simulink model "F16ASYM_Controlled_AoA"  (R2012b)
settings: Solver=ode3  SolverMode=SingleTasking  StartTime=0.0  StopTime=inf  FixedStep=T_sim  RelTol=1e-3
InitFcn:
  | load('NN_c_weights_Last_stable.mat')
values from neighbouring files (symbols this model uses):
  K_b_AoA = params(3)    [Cost_function.m]
  K_b_q = params(4)    [Cost_function.m]
  learning = 20    [Scheduling_desing.m]
  Model_used_flag = 1    [Scheduling_desing.m]
  reg_param = 0.5    [Scheduling_desing.m]
  T_sim = 0.02    [Scheduling_desing.m]
  tau_AoA = params(1)    [Cost_function.m]
  tau_q = params(2)    [Cost_function.m]
  Theta_1_roll_last = [0.00183613313267 0.00115998993235 0.0006676025148 0.00194921904952 0.00134963559861 0.00034352059664 0.000447169388141 0.00146749660935 0.00110199952389 7.77922383894e-05 0.00109492833348 0.00192687590535 ... (360 elements, 30x12)]    [NN_i_weights_LAST_STABLE.mat]
  Theta_2_roll_last = [0.000469743069697 0.000355923851088 0.00180035760697 0.00191855117771 0.00118851504447 0.0013331642065 0.0013164316578 0.000643981263341 0.00176817665434 0.000113802099363 0.000426534542462 0.00113815782354 ... (620 elements, 20x31)]    [NN_i_weights_LAST_STABLE.mat]
  Theta_3_roll_last = [9.62071520568e-05 -0.000389870886846 2.08260845013e-05 0.000140787743673 -0.000917525755397 -0.0014324207578 -0.00154701573815 -0.00131544476264 -0.00101205584381 5.06515794689e-05 -0.00111443483676 -0.00143957416141 ... (21 elements, 1x21)]    [NN_i_weights_LAST_STABLE.mat]
  V_long_lastA_w_z = [0.352826086601 -0.253633004548 -0.642535042878 0.237749930435 -0.618390629538 0.858074761295 0.268211230628 -0.448715080196 -0.0406384631192 0.401147605577 0.60598427709 0.0500551915851 ... (300 elements, 30x10)]    [NN_i_weights_LAST_STABLE.mat]
  V_long_lastAoA = [0.0774300162379 0.0911421319631 0.0352371192557 0.0542170286952 0.0651171200844 0.0177112012707 0.0982957728448 0.000259994642558 0.0194724569123 0.0466321328252 0.0556687953852 0.0252668067142 ... (300 elements, 30x10)]    [NN_i_weights_LAST_STABLE.mat]
  V_roll_last = [0.0540918675943 0.0557493347212 0.0839792276608 0.0460576391794 0.0671229058124 0.100220403067 0.0722493281881 0.0648875457457 0.00447599349201 0.0607299103823 0.0488037966361 0.0176785979393 ... (360 elements, 30x12)]    [NN_i_weights_LAST_STABLE.mat]
  V_yaw_last = [0.0965149149679 0.00833616709545 0.0365734360076 0.0523944217566 0.00790252078455 0.0700053845887 0.0345164868709 0.0111568465295 0.094060639546 0.0205483560006 0.000798047494256 0.0862769385758 ... (360 elements, 30x12)]    [NN_i_weights_LAST_STABLE.mat]
  velocity = M_eval_sche(I,J)*a    [Scheduling_desing.m]
  W_long_lastA_w_z = [-0.0522913429974 0.00385484301394 -0.00465489482472 -0.0139416219936 0.00295196421483 -0.013027768541 0.00585545058915 0.00278802233571 -0.00906272782329 -0.000396112031465 0.00405849743321 0.00509668457818 ... (31 elements, 1x31)]    [NN_i_weights_LAST_STABLE.mat]
  W_long_lastAoA = [-0.0192589013922 0.00873109909713 0.00432649597332 0.0420946902441 0.0293366820194 0.0351497798191 0.0234952374236 0.0360841187718 0.0112233388211 0.030147202199 0.0369533138617 0.00218839076415 ... (31 elements, 1x31)]    [NN_i_weights_LAST_STABLE.mat]
  W_roll_last = [-0.0006515532842 0.000535485585715 0.000550946920743 0.000806030945453 0.00045976209382 0.00065557954304 0.000945902185602 0.00070191398535 0.000635215543728 4.66501377412e-05 0.000597079583757 0.000485790566765 ... (31 elements, 1x31)]    [NN_i_weights_LAST_STABLE.mat]
  W_yaw_last = [-4.34263633305e-05 8.83823048922e-05 1.65575463724e-05 3.60293102233e-05 5.19752447623e-05 7.06399280852e-06 7.02425975821e-05 3.62680255076e-05 1.29996379937e-05 8.05072914397e-05 2.39941870661e-05 2.52427840574e-06 ... (31 elements, 1x31)]    [NN_i_weights_LAST_STABLE.mat]
undefined symbols (not defined in the file or in its folder): a1, alpha_map_eval, B, beta_map_eval, C_L_0, DiscIntNeverNeededParam, fi_flag_Simulink, G_eval, H_sq, H_sq_autotrim, k_B, m_B, M_sq, M_sq_autotrim, sigbuilder_block, Stall_curve, trim_control, trim_state, trim_throttle, V_Comp_A_w_z_last, V_Comp_last, V_roll_lastMOD, W_Comp_A_w_z_last, W_Comp_last, W_roll_lastMOD
libraries: Adaptive_FaultTolerantControl x43, dspsigops x29, F16_Actuator_Library x14, simulink x8, aerolibatmos2 x7, dsparch4 x6, simulink_extras x5, aerolibtransform2 x5, qcatlib x4, dspmtrx3 x3, dspvision x2, dspsnks4 x2
(part 2 of 11)

== system F16ASYM_Controlled_AoA/Anti-windup Calculation/Anti-windup: Reconfigurable ==
  note: INPUTS
      | States:
      |
      | 1. Altitude
      | 2. TAS velocity
      | 3. alpha in rad
      | 4. beta in rads
      | 5. P
      | 6. Q
      | 7. R
      | 8. Throttle
      | 9. Elevator_L in deg
      | 10. Elevator_R in deg
      | 11. Aileron_L
      | 12. Aileron_R
      | 13. Rudder
      | 14. LEF_L
      | 15. LEF_R
      |
      | RECONFIGURATION PARAMETERS
      |
      | 16. mass  Estimated mass
      | 17. S_current_L
      | 18. S_current_R
      | 19. S_fin_current
      | 20. x_cg
      | 21. Jy
      | 22. Jxz
      | 23. Jz
      | 24. Jx
      | 25. EFF_el_L
      | 26. EFF_el_R
      | 27. EFF_ail_L
      | 28 EFF_ail_R
      | 29. EFF_rud
      | 30. EFF_lef_L
      | 31. EFF_lef_R
      | 32. Delta_C_Lift_X
      | 33. Delta_C_Drag_X
      | 34. Delta_C_m_X
  note: Reached Angular accel
  note: Converto to Angular accelerations
  Ang accel comm : Inport
  Est reconf : Inport  Port=2
  All_meas : Inport  Port=3
  Surf saturated : Inport  Port=4
  Control_defl : Inport  Port=5
  AWU signals : Scope
      settings: YMin=-2.5  YMax=4.5  SaveName=ScopeData7
  AWU signals1 : Scope
      settings: YMin=-3.5  YMax=1.5  SaveName=ScopeData12
  Analog Filter Design1 : dsparch4/Analog Filter Design  method=Butterworth  filttype=Lowpass  N=8  Wlo=2*pi/T_sim/5  Whi=80  Rp=2  Rs=40
  Analog Filter Design2 : dsparch4/Analog Filter Design  method=Butterworth  filttype=Lowpass  N=8  Wlo=2*pi/T_sim/5  Whi=80  Rp=2  Rs=40
  Analog Filter Design3 : dsparch4/Analog Filter Design  method=Butterworth  filttype=Lowpass  N=8  Wlo=2*pi/T_sim/5  Whi=80  Rp=2  Rs=40
  Ang Accel : MATLAB Function
  Antiwindup calculation : MATLAB Function  TreatAsAtomicUnit=on
  Bus Selector : BusSelector  OutputSignals=signal1.Alt meas (m),signal1.V_TAS (m/s),signal1.AoA meas (rad),signal1.SS meas (rad),signal1.omega_b meas (rad/s),signal1.Throttle_meas
  Bus Selector1 : BusSelector  OutputSignals=signal2.q (Pa),signal1.omega_b meas (rad/s)
  Bus Selector2 : BusSelector  OutputSignals=Reconfig signal
  Demux : Demux  Outputs=3
  Demux1 : Demux  Outputs=3
  Effectiveness Matrix B : Constant  Value=B
  Memory1 : Memory  X0=[0,0,0]
  "Mom coefficients that can was reached " : MATLABFcn  MATLABFcn=Moms_Coeff_Reconf_estimator  OutputDimensions=3  OutputSignalType=real
  Moments : Subsystem
  Mux : Mux  Inputs=3
  Mux1 : Mux  Inputs=7
  Mux2 : Mux  Inputs=3
  Mux3 : Mux  Inputs=[15 19]
  Selector : Selector  InputPortWidth=8  IndexOptions=Index vector (dialog)  Indices=1:7  OutputSizes=1
  Signal Specification : SignalSpecification  Dimensions=19
  Transfer Fcn1 : TransferFcn  Commented=on  Numerator=10  Denominator=[1 10]
  Anti-windup signals : Outport
  wires:
  Bus Selector/6 -> Mux1/6  "<Throttle_meas>"
  Control_defl/1 -> Selector/1
  Bus Selector/4 -> Mux1/4  "<SS meas (rad)>"
  Bus Selector/3 -> Mux1/3  "<AoA meas (rad)>"
  Bus Selector/2 -> Mux1/2  "<V_TAS (m/s)>"
  Bus Selector/1 -> Mux1/1  "<Alt meas (m)>"
  Bus Selector/5 -> Mux1/5  "<omega_b meas (rad/s)>"
  Selector/1 -> Antiwindup calculation/5(deflections), Mux1/7
  Est reconf/1 -> Bus Selector2/1
  Bus Selector2/1 -> Signal Specification/1  "<Reconfig signal>"
  Mux1/1 -> Mux3/1
  Mux3/1 -> "Mom coefficients that can was reached "/1
  Signal Specification/1 -> Mux3/2
  All_meas/1 -> Bus Selector1/1, Bus Selector/1
  Ang Accel/2(q_dot) -> Mux/2
  Ang Accel/3(r_dot) -> Mux/3
  Ang Accel/1(p_dot) -> Mux/1
  Bus Selector1/2 -> Ang Accel/4(omega_b)  "<omega_b meas (rad/s)>"
  Moments/3(N) -> Ang Accel/3(N)
  Moments/2(M) -> Ang Accel/2(M)
  Moments/1(L) -> Ang Accel/1(L)
  Bus Selector1/1 -> Moments/4(q)  "<q (Pa)>"
  Demux/3 -> Moments/3(C_N)
  Demux/2 -> Moments/2(C_M)
  Demux/1 -> Moments/1(C_L)
  "Mom coefficients that can was reached "/1 -> Demux/1
  Mux/1 -> Antiwindup calculation/2(Ang_acell_achieved)
  Effectiveness Matrix B/1 -> Antiwindup calculation/4(B)
  Surf saturated/1 -> Antiwindup calculation/3(Saturations)
  Ang accel comm/1 -> Memory1/1
  Memory1/1 -> Antiwindup calculation/1(Ang_acell_comm)
  Antiwindup calculation/1(AWU) -> Demux1/1, AWU signals/1
  Demux1/1 -> Analog Filter Design3/1
  Demux1/2 -> Analog Filter Design1/1
  Analog Filter Design3/1 -> Mux2/1
  Analog Filter Design1/1 -> Mux2/2
  Analog Filter Design2/1 -> Mux2/3
  Demux1/3 -> Analog Filter Design2/1
  Mux2/1 -> AWU signals1/1, Anti-windup signals/1

== system F16ASYM_Controlled_AoA/Auto-trim, saturations sensibility and pilot help/Command A_w_z  or  A_gamma_z ==
  note: Pass this one if >0.5
  All meas : Inport
  Acc command : Inport  Port=2
  A_b : Product  Multiplication=Matrix(*)
  A_w : Product  Multiplication=Matrix(*)
  Bus Selector3 : BusSelector  OutputSignals=signal2.T_F_b->F_T,signal2.T_F_b->F_w
  Criteria : Constant  Value=Criteria
  Gain : Gain  Gain=[0;0;-1]
  Gain1 : Gain  Gain=-1
  Selector : Selector  InputPortWidth=3  IndexOptions=Index vector (dialog)  Indices=3  OutputSizes=1
  Switch : Switch  Threshold=0.5
  Transpose : dspmtrx3/Transpose  Hermitian=off  overflowFlag=off
  A_w_z : Outport
  wires:
  All meas/1 -> Bus Selector3/1
  Criteria/1 -> Switch/2
  Acc command/1 -> Switch/3, Gain/1
  Switch/1 -> A_w_z/1
  Bus Selector3/1 -> Transpose/1  "<T_F_b->F_T>"
  Transpose/1 -> A_b/1
  Gain/1 -> A_b/2
  Bus Selector3/2 -> A_w/1  "<T_F_b->F_w>"
  A_b/1 -> A_w/2
  A_w/1 -> Selector/1
  Selector/1 -> Gain1/1
  Gain1/1 -> Switch/1

== system F16ASYM_Controlled_AoA/Cockpit/Joystick ==
  Add1 : Sum
  Add2 : Sum
  Aileron : Selector  InputPortWidth=2  IndexOptions=Index vector (dialog)  Indices=1  OutputSizes=1
  Gain : Gain  Gain=0.01  OutDataTypeStr=double
  Gain{1..2,4,8} (4 alike) : Gain
  Gain3 : Gain  Gain=-1
  Gain5 : Gain  Gain=-10
  Gain6 : Gain  Gain=10  OutDataTypeStr=double
  Gain7 : Gain  Gain=-1
  Integrator Limited2 : Integrator  LimitOutput=on  UpperSaturationLimit=400  LowerSaturationLimit=-400
  Integrator Limited3 : Integrator  LimitOutput=on  UpperSaturationLimit=1  LowerSaturationLimit=-1
  Joystick Input : vrlib/Joystick Input  joyid=1  adjustports=on  forcefeed=off
  Manual Switch : ManualSwitch
  Selector1 : Selector  InputPortWidth=5  IndexOptions=Index vector (dialog)  Indices=1:2  OutputSizes=1
  Selector2 : Selector  InputPortWidth=5  IndexOptions=Index vector (dialog)  Indices=3  OutputSizes=1
  Selector3 : Selector  InputPortWidth=5  IndexOptions=Index vector (dialog)  Indices=4:5  OutputSizes=1
  Selector4 : Selector  InputPortWidth=10  IndexOptions=Index vector (dialog)  Indices=1  OutputSizes=1
  Selector5 : Selector  InputPortWidth=10  IndexOptions=Index vector (dialog)  Indices=4  OutputSizes=1
  Selector6 : Selector  InputPortWidth=10  IndexOptions=Index vector (dialog)  Indices=1  OutputSizes=1
  Selector7 : Selector  InputPortWidth=10  IndexOptions=Index vector (dialog)  Indices=4  OutputSizes=1
  elev : Selector  InputPortWidth=2  IndexOptions=Index vector (dialog)  Indices=2  OutputSizes=1
  speed des : Outport
  Throttle : Outport  Port=2
  Long: Acc : Outport  Port=3
  Roll : Outport  Port=4
  sideslip : Outport  Port=5
  wires:
  Integrator Limited3/1 -> Throttle/1  "Throttle"
  Aileron/1 -> Gain1/1
  Manual Switch/1 -> Aileron/1, elev/1
  Joystick Input/1 -> Selector2/1, Selector3/1, Selector1/1
  Selector1/1 -> Manual Switch/1
  Selector3/1 -> Manual Switch/2
  Selector4/1 -> Gain3/1
  Selector5/1 -> Gain4/1
  Gain3/1 -> Add1/1
  Gain4/1 -> Add1/2
  Add1/1 -> Gain/1
  Gain/1 -> Integrator Limited3/1
  elev/1 -> Gain2/1
  Gain1/1 -> Roll/1
  Selector2/1 -> Gain5/1
  Gain2/1 -> Long: Acc/1
  Gain5/1 -> sideslip/1
  Integrator Limited2/1 -> speed des/1  "Throttle"
  Joystick Input/2 -> Selector5/1, Selector7/1, Selector6/1, Selector4/1
  Selector6/1 -> Gain7/1
  Selector7/1 -> Gain8/1
  Gain7/1 -> Add2/1
  Gain8/1 -> Add2/2
  Add2/1 -> Gain6/1
  Gain6/1 -> Integrator Limited2/1

== system F16ASYM_Controlled_AoA/Cockpit/Signal Builder1 ==
  Demux : Demux  Tag=STV Demux
  FromWs : FromWorkspace  Tag=STV FromWs  VariableName=tuvar  SampleTime=0
      SigBuilderData=|
      | common.afterFinalStr = 'Extrapolate'
      | common.sampleTime = 0
      | dataSet.timeRange = [0 30]
      | dataSet.name = 'Group 1'
      | sbobj.Groups.Name = 'Group 1'
      | sbobj.Groups.Signals(1).Name = 'Signal 1'
      | sbobj.Groups.Signals(1).XData = [0 0.5 0.5 2.5 2.5 30]
      | sbobj.Groups.Signals(1).YData = [0 0 -1 -1 0 0]
      | sbobj.Groups.Signals(2).Name = 'Signal 5'
      | sbobj.Groups.Signals(2).XData = [0 4 4 6 6 30]
      | sbobj.Groups.Signals(2).YData = [0 0 1 1 0 0]
      | sbobj.Groups.Signals(3).Name = 'Signal 6'
      | sbobj.Groups.Signals(3).XData = [0 8 8 10 10 30]
      | sbobj.Groups.Signals(3).YData = [0 0 -0.5 -0.5 0 0]
      | sbobj.Groups.Signals(4).Name = 'Signal 7'
      | sbobj.Groups.Signals(4).XData = [0 12 12 14 14 30]
      | sbobj.Groups.Signals(4).YData = [0 0 0.5 0.5 0 0]
      | sbobj.Groups.TimeRange = [0 30]
  Signal 1 : Outport  Tag=STV Outport
  Signal 5 : Outport  Tag=STV Outport  Port=2
  Signal 6 : Outport  Tag=STV Outport  Port=3
  Signal 7 : Outport  Tag=STV Outport  Port=4
  wires:
  FromWs/1 -> Demux/1
  Demux/1 -> Signal 1/1
  Demux/2 -> Signal 5/1
  Demux/3 -> Signal 6/1
  Demux/4 -> Signal 7/1

== system F16ASYM_Controlled_AoA/Cockpit/Signal Builder2 ==
  Demux : Demux  Tag=STV Demux
  FromWs : FromWorkspace  Tag=STV FromWs  VariableName=tuvar  SampleTime=0
      SigBuilderData=|
      | common.afterFinalStr = 'Extrapolate'
      | common.sampleTime = 0
      | dataSet.timeRange = [0 10]
      | dataSet.name = 'Group 1'
      | sbobj.Groups.Name = 'Group 1'
      | sbobj.Groups.Signals(1).Name = 'Signal 1'
      | sbobj.Groups.Signals(1).XData = [0 5 5 8.02 8.02 10]
      | sbobj.Groups.Signals(1).YData = [0 0 -8.15 -8.15 0.64 0.7]
      | sbobj.Groups.Signals(2).Name = 'Signal 2'
      | sbobj.Groups.Signals(2).XData = [0 10]
      | sbobj.Groups.Signals(2).YData = [0 0]
      | sbobj.Groups.Signals(3).Name = 'Signal 3'
      | sbobj.Groups.Signals(3).XData = [0 10]
      | sbobj.Groups.Signals(3).YData = [0 0]
      | sbobj.Groups.Signals(4).Name = 'Signal 4'
      | sbobj.Groups.Signals(4).XData = [0 10]
      | sbobj.Groups.Signals(4).YData = [0 0]
  Signal 1 : Outport  Tag=STV Outport
  Signal 2 : Outport  Tag=STV Outport  Port=2
  Signal 3 : Outport  Tag=STV Outport  Port=3
  Signal 4 : Outport  Tag=STV Outport  Port=4
  wires:
  FromWs/1 -> Demux/1
  Demux/1 -> Signal 1/1
  Demux/2 -> Signal 2/1
  Demux/3 -> Signal 3/1
  Demux/4 -> Signal 4/1

== matlab function F16ASYM_Controlled_AoA/Anti-windup Calculation/Anti-windup: NO reconfigurable/Antiwindup calculation ==
  data: Ang_acell_comm input; AWU output; Ang_acell_achieved input; Saturations input; B input; deflections input
function AWU = AWU_calculation(Ang_acell_comm,Ang_acell_achieved,Saturations,B,deflections)
% Computing Saturation limits
sup_limit = [24,24,21,21,29,25,25]-1;
inf_limit = [-24,-24,-21,-21,-29,0,0]+1;

for i=1:7
    Saturations(i) = Saturation_smooth(abs(Saturations(i)),deflections(i),sup_limit(i),inf_limit(i));
end
Sat_B = B*Saturations;
B_max = B*ones(7,1);

AWU=zeros(3,1);

%% Method A
% % psi = 0.01; % % of the effort above the one we consider manouvreability is reduced
% % for i=1:3
% %     if i==1 && sign(deflections(3))== sign(deflections(4)) && abs(Sat_B(i))>psi*abs(B_max(i))
% %         AWU(2) = Ang_acell_comm(2) - Ang_acell_achieved(2); % we have to desaturate longitudinally not laterally
% %     elseif  i==1 && sign(deflections(3))~= sign(deflections(4)) && abs(Sat_B(i))>psi*abs(B_max(i))
% %         AWU(i) = Ang_acell_comm(i) - Ang_acell_achieved(i);
% %     elseif i~=1 && abs(Sat_B(i))>psi*abs(B_max(i))
% %         AWU(i) = Ang_acell_comm(i) - Ang_acell_achieved(i);
% %     end 
% % end

%% Method B
% % % % Long
% % % if Saturations(1)~=0 || Saturations(2)~=0 ||  Saturations(6)~=0 || Saturations(7)~=0 || ((Saturations(3)~=0 || Saturations(4)~=0) && sign(deflections(3))== sign(deflections(4)) ) 
% % %     AWU(2) = Ang_acell_comm(2) - Ang_acell_achieved(2);
% % % end
% % % % Lat-dir
% % % if ((Saturations(3)~=0 || Saturations(4)~=0) && sign(deflections(3)) ~= sign(deflections(4)) )  || Saturations(5)~=0 || Saturations(6)~=0 || Saturations(7)~=0
% % %     AWU(1) = Ang_acell_comm(1) - Ang_acell_achieved(1);
% % %     AWU(3) = Ang_acell_comm(3) - Ang_acell_achieved(3);
% % % 
% % % end



%% Method C
for i=1:3
        AWU(i) = (Ang_acell_comm(i) - Ang_acell_achieved(i))*Sat_B(i)/norm(B(i,:));
end

end

function Saturation_out = Saturation_smooth(Saturation,angle,sup_limit,inf_limit)

a=5;
Saturation_out  = ( 1 - 1./(1+exp(-a*(angle-inf_limit ))) + 1./(1+exp(-a*(angle-sup_limit ))) )*Saturation;


end

== matlab function F16ASYM_Controlled_AoA/Primary Controller/P  + Crossed NN + AWU+Lim + hand-over/P controller + adaptive Crossed NN + AWU+Lim   in AoA/Physical limitation/Ang Accel ==
  data: L input; p_dot output; q_dot output; r_dot output; M input; N input; omega_b input
function [p_dot,q_dot,r_dot] = Ang_accel(L,M,N,omega_b)
Jy  = 75673.6;
Jxz = 1331.4; 
Jz  = 85552.1;  
Jx  = 12874.8;
h_E = 216.9;

denom = Jx*Jz - Jxz*Jxz;

% % C1 = ((Jy - Jz)  * Jz  - (Jxz * Jxz))/ Gamma;
% % C2 = ((Jx - Jy + Jz ) * Jxz ) / Gamma;
% % C3 = Jz / Gamma;
% % C4 = Jxz / Gamma;
% % C5 = (Jz - Jx) / Jy;
% % C6 = Jxz / Jy ;
% % C7 = 1 / Jy;
% % C8 = (Jx * (Jx - Jy ) + Jxz * Jxz) / Gamma;
% % C9 = Jx / Gamma;


p_dot =  (Jz*L + Jxz*N - (Jz*(Jz-Jy)+Jxz*Jxz)*omega_b(2)*omega_b(3) + Jxz*(Jx-Jy+Jz)*omega_b(1)*omega_b(2) + Jxz*omega_b(2)*h_E)/denom;

q_dot = (M + (Jz-Jx)*omega_b(1)*omega_b(3) - Jxz*(omega_b(1)*omega_b(1)-omega_b(3)*omega_b(3)) - omega_b(3)*h_E)/Jy;


r_dot = (Jx*N + Jxz*L + (Jx*(Jx-Jy)+Jxz*Jxz)*omega_b(1)*omega_b(2) - Jxz*(Jx-Jy+Jz)*omega_b(2)*omega_b(3) +  Jx*omega_b(2)*h_E)/denom;

== matlab function F16ASYM_Controlled_AoA/Primary Controller/P  + Crossed NN + AWU+Lim + hand-over/P controller + adaptive Crossed NN + AWU+Lim    in ACC /Physical limitation/max deflections estimator ==
  data: v_comm input; max_defl output; B parameter
function max_defl = Max_defl(v_comm,B)
sup_limit = [24,24,21,21,29,25,25];
inf_limit = [-24,-24,-21,-21,-29,0,0];

def=B;
for i=1:3
    def(i,:) = B(i,:).*sign(v_comm(i));
end
def_avg = mean(def,1);

max_defl = zeros(7,1);
for i=1:7
    if def_avg(1,i)>0
        max_defl(i) = sup_limit(i);
    else
        max_defl(i) = inf_limit(i);
    end
end

== matlab function F16ASYM_Controlled_AoA/P controller + adaptive Crossed NN + AWU+Lim+scheduling   in AoA/Physical limitation/max deflections estimator ==
  data: v_comm input; max_defl output; B parameter
function max_defl = Max_defl(v_comm,B)
sup_limit = [24,24,21,21,29,25,25];
inf_limit = [-24,-24,-21,-21,-29,0,0];

def=B;
for i=1:3
    def(i,:) = B(i,:).*sign(v_comm(i));
end
def_avg = mean(def,1);

max_defl = zeros(7,1);
for i=1:7
    if def_avg(1,i)>0
        max_defl(i) = sup_limit(i);
    else
        max_defl(i) = inf_limit(i);
    end
end

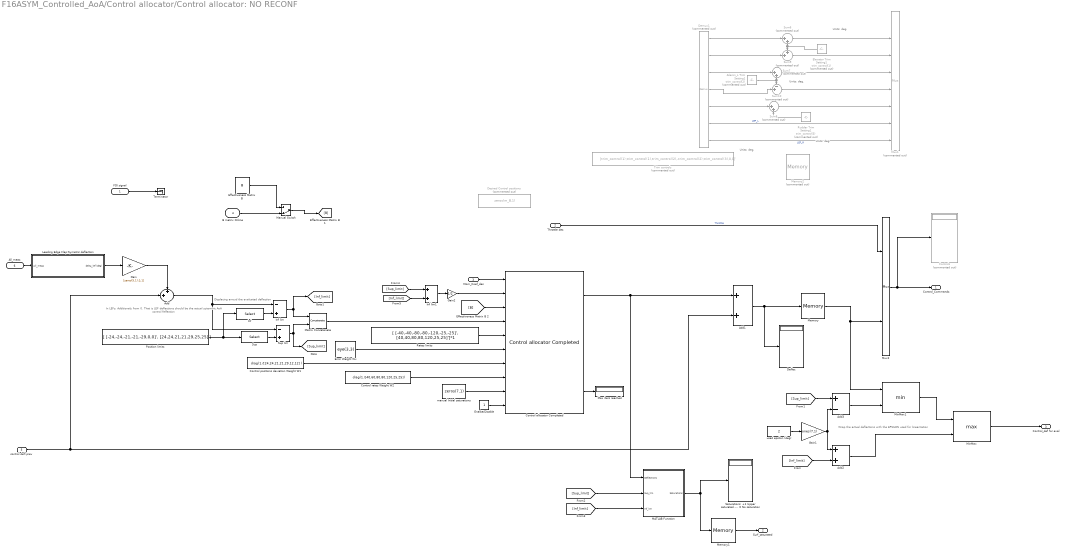
== system F16ASYM_Controlled_AoA/Control allocator/Control allocator: NO RECONF ==
  note: Wrap the actual deflections with the EPSILON
      |  used for linearization
  note: Units: deg.
  note: Units: deg.
  note: Units: deg.
  note: Units: deg.
  note: In LEFs: Additionaly from 0.  That is LEF deflections should be
      | the actual sytemtric AoA control felfection
  note: Displacing arroud the evaluated deflection
  FDI signal : Inport
  Throttle des : Inport  Port=2
  Mom_Coef_des : Inport  Port=3
  B matrix Online : Inport  Port=4
  control defl prev : Inport  Port=5
  All_meas : Inport  Port=6
  Add : Sum  Inputs=++|
  Add1 : Sum
  Add2 : Sum
  Add3 : Sum  Inputs=+-
  Aileron_L Trim Setting1 : Constant  Commented=on  Value=trim_control(2)
  "Control allocator Completed " : qcatlib/Control allocator Completed   alg=SLS  CA_type=QP  iter_max=100  gamma=1e6  k_B=3  m_B=7  T=T_sim  tol=1e-5
  Control positions deviation Weight W1 : Constant  Value=diag(1./[24,24,21,21,29,12,12] )
  Control rates Weight W2 : Constant  Value=diag(1./[40,60,80,80,120,25,25])
  Controls : Display  Commented=on
  Deflec : Display
  Demux1 : Demux  Commented=on  Outputs=[1,1,1,1,1,1,1]
  Desired Control positions : Constant  Commented=on  Value=zeros(m_B,1)
  Effectiveness Matrix B : Constant  Value=B
  Elevator Trim Setting1 : Constant  Commented=on  Value=trim_control(1)  VectorParams1D=off
  Enalbe/Disable : Constant
  Error Weight Wv : Constant  Value=eye(3,3)
  Gain : Gain  Gain=[zeros(5,1);1;1]
  Gain1 : Gain  Gain=ones(7,1)
  Gain2 : Gain  Gain=1/2
  Inf : Selector  NumberOfDimensions=2  InputPortWidth=3  IndexOptions=Index vector (dialog),Index vector (dialog)  Indices=[1:7],1  OutputSizes=1,1
  Inf lim : Sum  Inputs=-+
  Inf lim1 : Sum
  Leading Edge Flap:Symetric deflection : Subsystem
  MATLAB Function : MATLAB Function  TreatAsAtomicUnit=on
  Manual Switch : ManualSwitch  CurrentSetting=0
  Matrix Concatenate : Concatenate  Mode=Multidimensional array  ConcatenateDimension=2
  Max iters reached : Display
  Memory : Memory  X0=[trim_control(1),trim_control(1),trim_control(2),-trim_control(2),trim_control(3),0,0]'
  Memory1 : Memory  X0=zeros(7,1)
  Memory2 : Memory  Commented=on  X0=zeros(7,1)
  MinMax : MinMax  Function=max  Inputs=2
  MinMax1 : MinMax  Inputs=2
  Mux1 : Mux  Commented=on  Inputs=8
  Mux2 : Mux  Inputs=[1 7]
  Position limits : Constant  Value=[ [-24,-24,-21,-21,-29,0,0]', [24,24,21,21,29,25,25]']
  Rates limits : Constant  Value=[ [-40,-40,-80,-80,-120,-25,-25]', [40,40,80,80,120,25,25]']*1
  Rudder Trim Setting1 : Constant  Commented=on  Value=trim_control(3)
  Saturations: +1 Upper saturated -1 Lower saturated 0 No saturation : Display
  Sum10 : Sum  Commented=on  Inputs=-+|  SaturateOnIntegerOverflow=on  InputSameDT=on  OutDataTypeStr=Inherit: Same as first input
  Sum6 : Sum  Commented=on  Inputs=|++  SaturateOnIntegerOverflow=on  InputSameDT=on  OutDataTypeStr=Inherit: Same as first input
  Sum7 : Sum  Commented=on  Inputs=|++  SaturateOnIntegerOverflow=on  InputSameDT=on  OutDataTypeStr=Inherit: Same as first input
  Sum8 : Sum  Commented=on  Inputs=|++  SaturateOnIntegerOverflow=on  InputSameDT=on  OutDataTypeStr=Inherit: Same as first input
  Sum9 : Sum  Commented=on  Inputs=++|  SaturateOnIntegerOverflow=on  InputSameDT=on  OutDataTypeStr=Inherit: Same as first input
  Sup : Selector  NumberOfDimensions=2  InputPortWidth=3  IndexOptions=Index vector (dialog),Index vector (dialog)  Indices=[1:7],2  OutputSizes=1,1
  Sup lim : Sum  Inputs=-+
  Terminator : Terminator
  "Trim controls " : Constant  Commented=on  Value=[trim_control(1),trim_control(1),trim_control(2),-trim_control(2),trim_control(3),0,0]'
  manual Initial saturations : Constant  Value=zeros(7,1)
  used epsilon (deg) : Constant  Value=2
  Control_Commands : Outport
  Surf_saturated : Outport  Port=2
  Control_def for eval : Outport  Port=3
  wires:
  MinMax/1 -> Control_def for eval/1
  MinMax1/1 -> MinMax/1
  Add3/1 -> MinMax1/2
  used epsilon (deg)/1 -> Gain1/1
  [Inf_limit] -> Add2/2
  Gain1/1 -> Add3/2, Add2/1
  [Sup_limit] -> Add3/1
  Add2/1 -> MinMax/2
  Memory/1 -> Mux2/2, MinMax1/1
  Add1/1 -> Memory/1, Deflec/1
  Demux1/5 -> Sum8/1
  Rudder Trim Setting1/1 -> Sum8/2
  Elevator Trim Setting1/1 -> Sum9/1, Sum6/2
  Demux1/4 -> Sum10/2
  Demux1/3 -> Sum7/1
  Demux1/2 -> Sum9/2
  Demux1/1 -> Sum6/1
  Demux1/7 -> Mux1/8  "LEF_R"
  Demux1/6 -> Mux1/7  "LEF_L"
  Sum9/1 -> Mux1/3
  Sum6/1 -> Mux1/2
  Aileron_L Trim Setting1/1 -> Sum10/1, Sum7/2
  Sum10/1 -> Mux1/5
  Sum8/1 -> Mux1/6
  Sum7/1 -> Mux1/4
  ? -> Mux1/1  "Throttle"
  Control positions deviation Weight W1/1 -> "Control allocator Completed "/7
  FDI signal/1 -> Terminator/1
  Leading Edge Flap:Symetric deflection/1(delta_lef (deg)) -> Gain/1
  All_meas/1 -> Leading Edge Flap:Symetric deflection/1(All_meas)
  Gain/1 -> Add/1
  control defl prev/1 -> Add1/2, Add/2
  Manual Switch/1 -> [B]
  Effectiveness Matrix B/1 -> Manual Switch/1
  B matrix Online/1 -> Manual Switch/2
  "Control allocator Completed "/1 -> MATLAB Function/1(Deflections), Add1/1
  Enalbe/Disable/1 -> "Control allocator Completed "/10
  manual Initial saturations/1 -> "Control allocator Completed "/9
  "Control allocator Completed "/3 -> Max iters reached/1
  [B] -> "Control allocator Completed "/3
  Sup lim/1 -> [Sup_limit], Matrix Concatenate/2
  Inf lim/1 -> [Inf_limit], Matrix Concatenate/1
  Matrix Concatenate/1 -> "Control allocator Completed "/4
  Inf/1 -> Inf lim/2
  Add/1 -> Inf lim/1, Sup lim/1
  Sup/1 -> Sup lim/2
  Control rates Weight W2/1 -> "Control allocator Completed "/8
  Error Weight Wv/1 -> "Control allocator Completed "/6
  Rates limits/1 -> "Control allocator Completed "/5
  Position limits/1 -> Sup/1, Inf/1
  Gain2/1 -> "Control allocator Completed "/2
  Mux2/1 -> Control_Commands/1, Controls/1
  Throttle des/1 -> Mux2/1  "Throttle"
  Mom_Coef_des/1 -> "Control allocator Completed "/1
  [Sup_limit] -> MATLAB Function/2(Sup_lim)
  [Inf_limit] -> MATLAB Function/3(Inf_lim)
  MATLAB Function/1(Saturations) -> Memory1/1, Saturations: +1 Upper saturated -1 Lower saturated 0 No saturation/1
  [Sup_limit] -> Inf lim1/1
  [Inf_limit] -> Inf lim1/2
  Inf lim1/1 -> Gain2/1
  Memory1/1 -> Surf_saturated/1

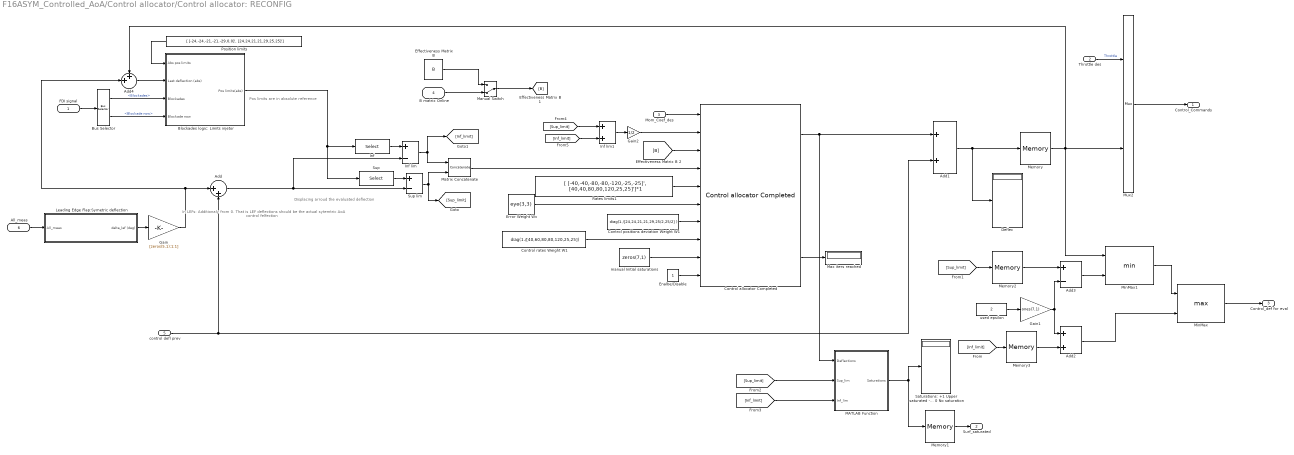
== system F16ASYM_Controlled_AoA/Control allocator/Control allocator: RECONFIG ==
  note: Pos limits are in absolute reference
  note: In LEFs: Additionaly from 0.  That is LEF deflections should be
      | the actual sytemtric AoA control felfection
  note: Displacing arroud the evaluated deflection
  FDI signal : Inport
  Throttle des : Inport  Port=2
  Mom_Coef_des : Inport  Port=3
  B matrix Online : Inport  Port=4
  control defl prev : Inport  Port=5
  All_meas : Inport  Port=6
  Add : Sum  Inputs=|++
  Add1 : Sum
  Add2 : Sum
  Add3 : Sum  Inputs=+-
  Add4 : Sum  Inputs=++|
  Blockades logic: Limits injetor : Subsystem
  Bus Selector : BusSelector  OutputSignals=Blockades,Blockade now
  "Control allocator Completed " : qcatlib/Control allocator Completed   alg=WLS  CA_type=QP  iter_max=100  gamma=1e8  k_B=3  m_B=7  T=T_sim  tol=1e-5
  Control positions deviation Weight W1 : Constant  Value=diag(1./[24,24,21,21,29,25/2,25/2] )
  Control rates Weight W1 : Constant  Value=diag(1./[40,60,80,80,120,25,25])
  Deflec : Display
  Effectiveness Matrix B : Constant  Value=B
  Enalbe/Disable : Constant
  Error Weight Wv : Constant  Value=eye(3,3)
  Gain : Gain  Gain=[zeros(5,1);1;1]
  Gain1 : Gain  Gain=ones(7,1)
  Gain2 : Gain  Gain=1/2
  Inf : Selector  NumberOfDimensions=2  InputPortWidth=3  IndexOptions=Index vector (dialog),Index vector (dialog)  Indices=[1:7],1  OutputSizes=1,1
  Inf lim : Sum  Inputs=+-
  Inf lim1 : Sum
  Leading Edge Flap:Symetric deflection : Subsystem
  MATLAB Function : MATLAB Function  TreatAsAtomicUnit=on
  Manual Switch : ManualSwitch  CurrentSetting=0
  Matrix Concatenate : Concatenate  Mode=Multidimensional array  ConcatenateDimension=2
  Max iters reached : Display
  Memory : Memory  X0=[trim_control(1),trim_control(1),trim_control(2),-trim_control(2),trim_control(3),0,0]'
  Memory1 : Memory  X0=zeros(7,1)
  Memory2 : Memory  X0=[24,24,21,21,29,25,25]'
  Memory3 : Memory  X0=[-24,-24,-21,-21,-29,0,0]'
  MinMax : MinMax  Function=max  Inputs=2
  MinMax1 : MinMax  Inputs=2
  Mux2 : Mux  Inputs=[1 7]
  Position limits : Constant  Value=[ [-24,-24,-21,-21,-29,0,0]', [24,24,21,21,29,25,25]']
  Rates limits1 : Constant  Value=[ [-40,-40,-80,-80,-120,-25,-25]', [40,40,80,80,120,25,25]']*1
  Saturations: +1 Upper saturated -1 Lower saturated 0 No saturation : Display
  Sup : Selector  NumberOfDimensions=2  InputPortWidth=3  IndexOptions=Index vector (dialog),Index vector (dialog)  Indices=[1:7],2  OutputSizes=1,1
  Sup lim : Sum  Inputs=+-
  manual Initial saturations : Constant  Value=zeros(7,1)
  used epsilon : Constant  Value=2
  Control_Commands : Outport
  Surf_saturated : Outport  Port=2
  Control_def for eval : Outport  Port=3
  wires:
  Mom_Coef_des/1 -> "Control allocator Completed "/1
  Throttle des/1 -> Mux2/1  "Throttle"
  Mux2/1 -> Control_Commands/1
  Rates limits1/1 -> "Control allocator Completed "/5
  Error Weight Wv/1 -> "Control allocator Completed "/6
  Control rates Weight W1/1 -> "Control allocator Completed "/8
  Sup/1 -> Sup lim/1
  Add/1 -> Inf lim/2, Sup lim/2
  Inf/1 -> Inf lim/1
  Matrix Concatenate/1 -> "Control allocator Completed "/4
  Inf lim/1 -> Matrix Concatenate/1, [Inf_limit]
  Sup lim/1 -> Matrix Concatenate/2, [Sup_limit]
  [B] -> "Control allocator Completed "/3
  "Control allocator Completed "/3 -> Max iters reached/1
  manual Initial saturations/1 -> "Control allocator Completed "/9
  Enalbe/Disable/1 -> "Control allocator Completed "/10
  B matrix Online/1 -> Manual Switch/2
  Effectiveness Matrix B/1 -> Manual Switch/1
  control defl prev/1 -> Add1/2, Add/2
  Gain/1 -> Add/1, Add4/2
  All_meas/1 -> Leading Edge Flap:Symetric deflection/1(All_meas)
  Leading Edge Flap:Symetric deflection/1(delta_lef (deg)) -> Gain/1
  Control positions deviation Weight W1/1 -> "Control allocator Completed "/7
  Add1/1 -> Deflec/1, Memory/1
  Memory/1 -> MinMax1/1, Mux2/2, Add4/1
  Add2/1 -> MinMax/2
  [Sup_limit] -> Memory2/1
  Gain1/1 -> Add2/1, Add3/2
  [Inf_limit] -> Memory3/1
  used epsilon/1 -> Gain1/1
  Add3/1 -> MinMax1/2
  MinMax1/1 -> MinMax/1
  MinMax/1 -> Control_def for eval/1
  Blockades logic: Limits injetor/1(Pos limits(abs)) -> Inf/1, Sup/1
  Bus Selector/1 -> Blockades logic: Limits injetor/3(Blockades)  "<Blockades>"
  Bus Selector/2 -> Blockades logic: Limits injetor/4(Blockade now)  "<Blockade now>"
  FDI signal/1 -> Bus Selector/1
  Add4/1 -> Blockades logic: Limits injetor/2(Last deflection (abs))
  Position limits/1 -> Blockades logic: Limits injetor/1(Abs pos limits)
  Manual Switch/1 -> [B]
  [Sup_limit] -> Inf lim1/1
  [Inf_limit] -> Inf lim1/2
  Inf lim1/1 -> Gain2/1
  Gain2/1 -> "Control allocator Completed "/2
  "Control allocator Completed "/1 -> Add1/1, MATLAB Function/1(Deflections)
  [Sup_limit] -> MATLAB Function/2(Sup_lim)
  [Inf_limit] -> MATLAB Function/3(Inf_lim)
  MATLAB Function/1(Saturations) -> Memory1/1, Saturations: +1 Upper saturated -1 Lower saturated 0 No saturation/1
  Memory1/1 -> Surf_saturated/1
  Memory2/1 -> Add3/1
  Memory3/1 -> Add2/2

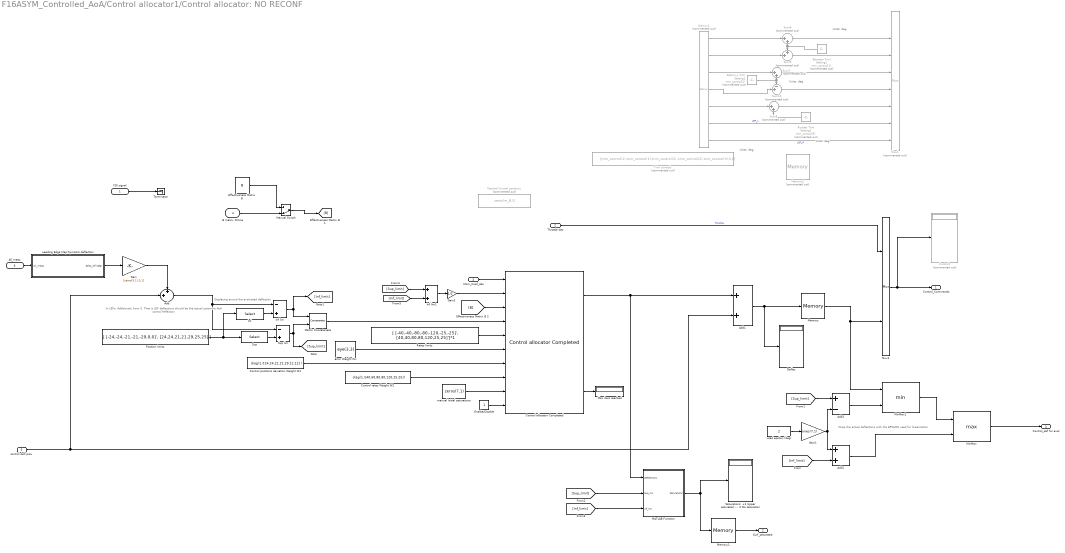
== system F16ASYM_Controlled_AoA/Control allocator1/Control allocator: NO RECONF ==
  note: Wrap the actual deflections with the EPSILON
      |  used for linearization
  note: Units: deg.
  note: Units: deg.
  note: Units: deg.
  note: Units: deg.
  note: In LEFs: Additionaly from 0.  That is LEF deflections should be
      | the actual sytemtric AoA control felfection
  note: Displacing arroud the evaluated deflection
  FDI signal : Inport
  Throttle des : Inport  Port=2
  Mom_Coef_des : Inport  Port=3
  B matrix Online : Inport  Port=4
  control defl prev : Inport  Port=5
  All_meas : Inport  Port=6
  Add : Sum  Inputs=++|
  Add1 : Sum
  Add2 : Sum
  Add3 : Sum  Inputs=+-
  Aileron_L Trim Setting1 : Constant  Commented=on  Value=trim_control(2)
  "Control allocator Completed " : qcatlib/Control allocator Completed   alg=SLS  CA_type=QP  iter_max=100  gamma=1e6  k_B=3  m_B=7  T=T_sim  tol=1e-5
  Control positions deviation Weight W1 : Constant  Value=diag(1./[24,24,21,21,29,12,12] )
  Control rates Weight W2 : Constant  Value=diag(1./[40,60,80,80,120,25,25])
  Controls : Display  Commented=on
  Deflec : Display
  Demux1 : Demux  Commented=on  Outputs=[1,1,1,1,1,1,1]
  Desired Control positions : Constant  Commented=on  Value=zeros(m_B,1)
  Effectiveness Matrix B : Constant  Value=B
  Elevator Trim Setting1 : Constant  Commented=on  Value=trim_control(1)  VectorParams1D=off
  Enalbe/Disable : Constant
  Error Weight Wv : Constant  Value=eye(3,3)
  Gain : Gain  Gain=[zeros(5,1);1;1]
  Gain1 : Gain  Gain=ones(7,1)
  Gain2 : Gain  Gain=1/2
  Inf : Selector  NumberOfDimensions=2  InputPortWidth=3  IndexOptions=Index vector (dialog),Index vector (dialog)  Indices=[1:7],1  OutputSizes=1,1
  Inf lim : Sum  Inputs=-+
  Inf lim1 : Sum
  Leading Edge Flap:Symetric deflection : Subsystem
  MATLAB Function : MATLAB Function  TreatAsAtomicUnit=on
  Manual Switch : ManualSwitch  CurrentSetting=0
  Matrix Concatenate : Concatenate  Mode=Multidimensional array  ConcatenateDimension=2
  Max iters reached : Display
  Memory : Memory  X0=[trim_control(1),trim_control(1),trim_control(2),-trim_control(2),trim_control(3),0,0]'
  Memory1 : Memory  X0=zeros(7,1)
  Memory2 : Memory  Commented=on  X0=zeros(7,1)
  MinMax : MinMax  Function=max  Inputs=2
  MinMax1 : MinMax  Inputs=2
  Mux1 : Mux  Commented=on  Inputs=8
  Mux2 : Mux  Inputs=[1 7]
  Position limits : Constant  Value=[ [-24,-24,-21,-21,-29,0,0]', [24,24,21,21,29,25,25]']
  Rates limits : Constant  Value=[ [-40,-40,-80,-80,-120,-25,-25]', [40,40,80,80,120,25,25]']*1
  Rudder Trim Setting1 : Constant  Commented=on  Value=trim_control(3)
  Saturations: +1 Upper saturated -1 Lower saturated 0 No saturation : Display
  Sum10 : Sum  Commented=on  Inputs=-+|  SaturateOnIntegerOverflow=on  InputSameDT=on  OutDataTypeStr=Inherit: Same as first input
  Sum6 : Sum  Commented=on  Inputs=|++  SaturateOnIntegerOverflow=on  InputSameDT=on  OutDataTypeStr=Inherit: Same as first input
  Sum7 : Sum  Commented=on  Inputs=|++  SaturateOnIntegerOverflow=on  InputSameDT=on  OutDataTypeStr=Inherit: Same as first input
  Sum8 : Sum  Commented=on  Inputs=|++  SaturateOnIntegerOverflow=on  InputSameDT=on  OutDataTypeStr=Inherit: Same as first input
  Sum9 : Sum  Commented=on  Inputs=++|  SaturateOnIntegerOverflow=on  InputSameDT=on  OutDataTypeStr=Inherit: Same as first input
  Sup : Selector  NumberOfDimensions=2  InputPortWidth=3  IndexOptions=Index vector (dialog),Index vector (dialog)  Indices=[1:7],2  OutputSizes=1,1
  Sup lim : Sum  Inputs=-+
  Terminator : Terminator
  "Trim controls " : Constant  Commented=on  Value=[trim_control(1),trim_control(1),trim_control(2),-trim_control(2),trim_control(3),0,0]'
  manual Initial saturations : Constant  Value=zeros(7,1)
  used epsilon (deg) : Constant  Value=2
  Control_Commands : Outport
  Surf_saturated : Outport  Port=2
  Control_def for eval : Outport  Port=3
  wires:
  MinMax/1 -> Control_def for eval/1
  MinMax1/1 -> MinMax/1
  Add3/1 -> MinMax1/2
  used epsilon (deg)/1 -> Gain1/1
  [Inf_limit] -> Add2/2
  Gain1/1 -> Add3/2, Add2/1
  [Sup_limit] -> Add3/1
  Add2/1 -> MinMax/2
  Memory/1 -> Mux2/2, MinMax1/1
  Add1/1 -> Memory/1, Deflec/1
  Demux1/5 -> Sum8/1
  Rudder Trim Setting1/1 -> Sum8/2
  Elevator Trim Setting1/1 -> Sum9/1, Sum6/2
  Demux1/4 -> Sum10/2
  Demux1/3 -> Sum7/1
  Demux1/2 -> Sum9/2
  Demux1/1 -> Sum6/1
  Demux1/7 -> Mux1/8  "LEF_R"
  Demux1/6 -> Mux1/7  "LEF_L"
  Sum9/1 -> Mux1/3
  Sum6/1 -> Mux1/2
  Aileron_L Trim Setting1/1 -> Sum10/1, Sum7/2
  Sum10/1 -> Mux1/5
  Sum8/1 -> Mux1/6
  Sum7/1 -> Mux1/4
  ? -> Mux1/1  "Throttle"
  Control positions deviation Weight W1/1 -> "Control allocator Completed "/7
  FDI signal/1 -> Terminator/1
  Leading Edge Flap:Symetric deflection/1(delta_lef (deg)) -> Gain/1
  All_meas/1 -> Leading Edge Flap:Symetric deflection/1(All_meas)
  Gain/1 -> Add/1
  control defl prev/1 -> Add1/2, Add/2
  Manual Switch/1 -> [B]
  Effectiveness Matrix B/1 -> Manual Switch/1
  B matrix Online/1 -> Manual Switch/2
  "Control allocator Completed "/1 -> MATLAB Function/1(Deflections), Add1/1
  Enalbe/Disable/1 -> "Control allocator Completed "/10
  manual Initial saturations/1 -> "Control allocator Completed "/9
  "Control allocator Completed "/3 -> Max iters reached/1
  [B] -> "Control allocator Completed "/3
  Sup lim/1 -> [Sup_limit], Matrix Concatenate/2
  Inf lim/1 -> [Inf_limit], Matrix Concatenate/1
  Matrix Concatenate/1 -> "Control allocator Completed "/4
  Inf/1 -> Inf lim/2
  Add/1 -> Inf lim/1, Sup lim/1
  Sup/1 -> Sup lim/2
  Control rates Weight W2/1 -> "Control allocator Completed "/8
  Error Weight Wv/1 -> "Control allocator Completed "/6
  Rates limits/1 -> "Control allocator Completed "/5
  Position limits/1 -> Sup/1, Inf/1
  Gain2/1 -> "Control allocator Completed "/2
  Mux2/1 -> Control_Commands/1, Controls/1
  Throttle des/1 -> Mux2/1  "Throttle"
  Mom_Coef_des/1 -> "Control allocator Completed "/1
  [Sup_limit] -> MATLAB Function/2(Sup_lim)
  [Inf_limit] -> MATLAB Function/3(Inf_lim)
  MATLAB Function/1(Saturations) -> Memory1/1, Saturations: +1 Upper saturated -1 Lower saturated 0 No saturation/1
  [Sup_limit] -> Inf lim1/1
  [Inf_limit] -> Inf lim1/2
  Inf lim1/1 -> Gain2/1
  Memory1/1 -> Surf_saturated/1

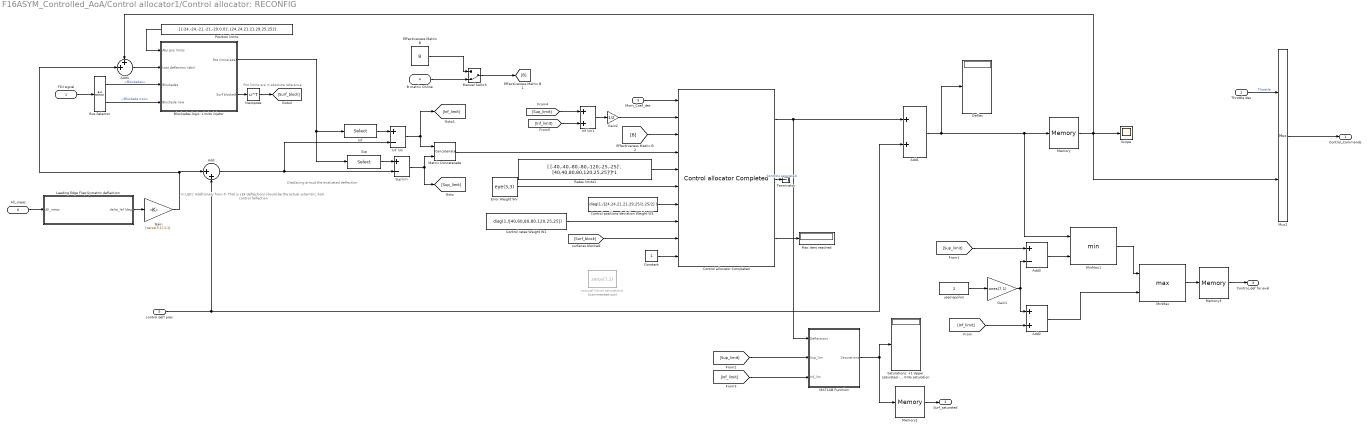
== system F16ASYM_Controlled_AoA/Control allocator1/Control allocator: RECONFIG ==
  note: Pos limits are in absolute reference
  note: In LEFs: Additionaly from 0.  That is LEF deflections should be
      | the actual sytemtric AoA control felfection
  note: Displacing arroud the evaluated deflection
  FDI signal : Inport
  Throttle des : Inport  Port=2
  Mom_Coef_des : Inport  Port=3
  B matrix Online : Inport  Port=4
  control defl prev : Inport  Port=5
  All_meas : Inport  Port=6
  Add : Sum  Inputs=|++
  Add1 : Sum  SampleTime=T_sim
  Add2 : Sum
  Add3 : Sum  Inputs=+-
  Add4 : Sum  Inputs=++|
  Blockades logic: Limits injetor : Subsystem
  Bus Selector : BusSelector  OutputSignals=Blockades,Blockade now
  Constant : Constant
  "Control allocator Completed " : qcatlib/Control allocator Completed   alg=WLS  CA_type=QP  iter_max=100  gamma=1e8  k_B=3  m_B=7  T=T_sim  tol=1e-5
  Control positions deviation Weight W1 : Constant  Value=diag(1./[24,24,21,21,29,25/2,25/2] )
  Control rates Weight W1 : Constant  Value=diag(1./[40,60,80,80,120,25,25])
  Deflec : Display
  Effectiveness Matrix B : Constant  Value=B
  Error Weight Wv : Constant  Value=eye(3,3)
  Gain : Gain  Gain=[zeros(5,1);1;1]
  Gain1 : Gain  Gain=ones(7,1)
  Gain2 : Gain  Gain=1/2
  Inf : Selector  NumberOfDimensions=2  InputPortWidth=3  IndexOptions=Index vector (dialog),Index vector (dialog)  Indices=[1:7],1  OutputSizes=1,1
  Inf lim : Sum  Inputs=+-
  Inf lim1 : Sum
  Leading Edge Flap:Symetric deflection : Subsystem
  MATLAB Function : MATLAB Function  TreatAsAtomicUnit=on
  Manual Switch : ManualSwitch  CurrentSetting=0
  Matrix Concatenate : Concatenate  Mode=Multidimensional array  ConcatenateDimension=2
  Max iters reached : Display
  Memory : Memory  X0=[trim_control(1),trim_control(1),trim_control(2),-trim_control(2),trim_control(3),0,0]'  InheritSampleTime=on
  Memory1 : Memory  X0=zeros(7,1)
  Memory3 : Memory  X0=[trim_control(1),trim_control(1),trim_control(2),-trim_control(2),trim_control(3),0,0]'  InheritSampleTime=on
  MinMax : MinMax  Function=max  Inputs=2
  MinMax1 : MinMax  Inputs=2
  Mux2 : Mux  Inputs=[1 7]
  Position limits : Constant  Value=[ [-24,-24,-21,-21,-29,0,0]', [24,24,21,21,29,25,25]']
  Rates limits1 : Constant  Value=[ [-40,-40,-80,-80,-120,-25,-25]', [40,40,80,80,120,25,25]']*1
  Saturations: +1 Upper saturated -1 Lower saturated 0 No saturation : Display
  Scope : Scope
      settings: YMin=-25  YMax=20  SaveName=ScopeData22
  Sup : Selector  NumberOfDimensions=2  InputPortWidth=3  IndexOptions=Index vector (dialog),Index vector (dialog)  Indices=[1:7],2  OutputSizes=1,1
  Sup lim : Sum  Inputs=+-
  Terminator : Terminator
  manual Initial saturations : Constant  Commented=on  Value=zeros(7,1)
  transpose : Math  Operator=transpose  SaturateOnIntegerOverflow=on
  used epsilon : Constant  Value=2
  Control_Commands : Outport
  Surf_saturated : Outport  Port=2
  Control_def for eval : Outport  Port=3
  wires:
  Mom_Coef_des/1 -> "Control allocator Completed "/1
  Throttle des/1 -> Mux2/1  "Throttle"
  Mux2/1 -> Control_Commands/1
  Rates limits1/1 -> "Control allocator Completed "/5
  Error Weight Wv/1 -> "Control allocator Completed "/6
  Control rates Weight W1/1 -> "Control allocator Completed "/8
  Sup/1 -> Sup lim/1
  Add/1 -> Inf lim/2, Sup lim/2
  Inf/1 -> Inf lim/1
  Matrix Concatenate/1 -> "Control allocator Completed "/4
  [B] -> "Control allocator Completed "/3
  "Control allocator Completed "/3 -> Max iters reached/1
  [Surf_block] -> "Control allocator Completed "/9
  Constant/1 -> "Control allocator Completed "/10
  B matrix Online/1 -> Manual Switch/2
  Effectiveness Matrix B/1 -> Manual Switch/1
  control defl prev/1 -> Add1/2, Add/2
  Gain/1 -> Add/1, Add4/2
  All_meas/1 -> Leading Edge Flap:Symetric deflection/1(All_meas)
  Leading Edge Flap:Symetric deflection/1(delta_lef (deg)) -> Gain/1
  Control positions deviation Weight W1/1 -> "Control allocator Completed "/7
  Add1/1 -> Deflec/1, MinMax1/1, Memory/1
  Add2/1 -> MinMax/2
  Gain1/1 -> Add2/1, Add3/2
  used epsilon/1 -> Gain1/1
  Add3/1 -> MinMax1/2
  MinMax1/1 -> MinMax/1
  MinMax/1 -> Memory3/1
  Bus Selector/1 -> Blockades logic: Limits injetor/3(Blockades)  "<Blockades>"
  Bus Selector/2 -> Blockades logic: Limits injetor/4(Blockade now)  "<Blockade now>"
  FDI signal/1 -> Bus Selector/1
  Add4/1 -> Blockades logic: Limits injetor/2(Last deflection (abs))
  Position limits/1 -> Blockades logic: Limits injetor/1(Abs pos limits)
  Manual Switch/1 -> [B]
  [Sup_limit] -> Inf lim1/1
  [Inf_limit] -> Inf lim1/2
  Inf lim1/1 -> Gain2/1
  Gain2/1 -> "Control allocator Completed "/2
  "Control allocator Completed "/1 -> Add1/1, MATLAB Function/1(Deflections)
  [Sup_limit] -> MATLAB Function/2(Sup_lim)
  [Inf_limit] -> MATLAB Function/3(Inf_lim)
  MATLAB Function/1(Saturations) -> Memory1/1, Saturations: +1 Upper saturated -1 Lower saturated 0 No saturation/1
  Memory1/1 -> Surf_saturated/1
  "Control allocator Completed "/2 -> Terminator/1  "Controls saturated"
  Memory/1 -> Mux2/2, Scope/1, Add4/1
  Blockades logic: Limits injetor/2(Surf blocked) -> transpose/1
  transpose/1 -> [Surf_block]
  Sup lim/1 -> [Sup_limit], Matrix Concatenate/2
  Inf lim/1 -> [Inf_limit], Matrix Concatenate/1
  [Inf_limit] -> Add2/2
  [Sup_limit] -> Add3/1
  Memory3/1 -> Control_def for eval/1
  Blockades logic: Limits injetor/1(Pos limits(abs)) -> Inf/1, Sup/1

== system F16ASYM_Controlled_AoA/Environment params Estimations/Mach number ==
  V : Inport
  a : Inport  Port=2
  Product1 : Product  Inputs=*/  SaturateOnIntegerOverflow=on  InputSameDT=on  OutDataTypeStr=Inherit: Same as first input
  Mach : Outport
  wires:
  Product1/1 -> Mach/1
  V/1 -> Product1/1
  a/1 -> Product1/2

== system F16ASYM_Controlled_AoA/F-16 Non-linear Plant/SYM and ASYM model: No reconfigurable ==
  note: Mdoel used  Flage tells the plant
      |  if Asymetric or symetric model is used:
      | 0: Symetric Model
      | 1: Asymetric model
  note: INPUTS
      | States:
      | 1. North Position
      | 2. East position
      | 3. Altitude
      | 4. Phi
      | 5. Theta
      | 6. Psi
      | 7. Total velocity
      | 8. alpha in rad
      | 9. beta in rads
      | 10. P
      | 11. Q
      | 12. R
      | 13. POW
      |
      | Controls:
      | 14. Throttle
      | 15. Elevator_L in deg
      | 16. Elevator_R in deg
      | 17. Aileron_L
      | 18. Aileron_R
      | 19. Rudder
      | 20. LEF_L
      | 21. LEF_R
      |
      | 22. Fidelity Flag
      |
      | 23. Model used: Asymetric or Symetric
  note: Fidelity Flage tells nlplant
      | which Model to use:
      | 0: Low Fidelity
      | 1: High Fidelity
  note: OUTPUTS
      | States:
      | 1. DEV North Position
      | 2. DEV East position
      | 3. DEV Altitude
      | 4.DEV  Phi
      | 5. DEV Theta
      | 6. DEV Psi
      | 7. DEV Total velocity
      | 8.DEV alpha in rad
      | 9.DEV  beta in rads
      | 10. DEV P
      | 11. DEV Q
      | 12. DEV R
      | 13. DEV POW
      |
      | Other outputs:
      | Accels of CG:
      | 14. anx_cg
      | 15. any_cg
      | 16. anz_cg
      | 17. mach
      | 18. qbar
      | 19. ps   Static Pressure
  note: Add the sytmetric deflection of the LEFs
  States : Inport
  Reconf params : Inport  Port=2
  Control Comands : Inport  Port=3
  Acels actual : Scope
      settings: YMin=-0.04  YMax=0.09  SaveName=ScopeData14
  Actuators Dynamcis : Subsystem  TreatAsAtomicUnit=on
  Bus Creator : BusCreator  Inputs=12
  Bus Creator1 : BusCreator  Inputs=2
  Demux : Demux  Outputs=[13 6]
  Demux1 : Demux  Outputs=8
  F16 nlsim nlplant Asymetrical : MATLABFcn  MATLABFcn=nlplantASYM  OutputDimensions=19  OutputSignalType=real
  Fidelity Flag : Constant  Value=fi_flag_Simulink
  Integrate F16 State Derivatives : Integrator  InitialCondition=trim_state
  Leading Edge Flap:Symetric deflection : Subsystem
  Model used flag : Constant  Value=Model_used_flag
  Mux1 : Mux  Inputs=8
  Mux5 : Mux  Inputs=[13 8 1 1]
  Rotation Angles to Direction Cosine Matrix : aerolibtransform2/Rotation Angles to Direction Cosine Matrix  rotationOrder=ZYX
  Selector : Selector  InputPortWidth=13  IndexOptions=Index vector (dialog)  Indices=[1:3]  OutputSizes=1
  Selector1 : Selector  InputPortWidth=13  IndexOptions=Index vector (dialog)  Indices=[1:3]  OutputSizes=1
  Selector2 : Selector  InputPortWidth=13  IndexOptions=Index vector (dialog)  Indices=[7]  OutputSizes=1
  Selector3 : Selector  InputPortWidth=13  IndexOptions=Index vector (dialog)  Indices=[8:9]  OutputSizes=1
  Selector4 : Selector  InputPortWidth=13  IndexOptions=Index vector (dialog)  Indices=[10:12]  OutputSizes=1
  Selector5 : Selector  InputPortWidth=13  IndexOptions=Index vector (dialog)  Indices=[4:6]  OutputSizes=1
  Selector6 : Selector  InputPortWidth=6  IndexOptions=Index vector (dialog)  Indices=[1:3]  OutputSizes=1
  Selector7 : Selector  InputPortWidth=3  IndexOptions=Index vector (dialog)  Indices=[3 2 1]  OutputSizes=1
  Selector9 : Selector  InputPortWidth=13  IndexOptions=Index vector (dialog)  Indices=[10:12]  OutputSizes=1
  Sum1 : Sum  Inputs=|++  SaturateOnIntegerOverflow=on  InputSameDT=on  OutDataTypeStr=Inherit: Same as first input
  Sum9 : Sum  Inputs=|++  SaturateOnIntegerOverflow=on  InputSameDT=on  OutDataTypeStr=Inherit: Same as first input
  Output_bus : Outport
  Actual control def : Outport  Port=2
  wires:
  Selector7/1 -> Rotation Angles to Direction Cosine Matrix/1
  Demux/2 -> Bus Creator/3, Selector6/1  "Other outs"
  Selector6/1 -> Bus Creator/11  "an_b_CG"
  Selector5/1 -> Bus Creator/9, Selector7/1  "euler"
  Selector4/1 -> Bus Creator/8  "p,q,r"
  Selector3/1 -> Bus Creator/7  "alpha,beta"
  Selector2/1 -> Bus Creator/6  "TAS"
  Selector1/1 -> Bus Creator/5  "V_e"
  Selector/1 -> Bus Creator/4  "X_e"
  Demux/1 -> Integrate F16 State Derivatives/1, Selector1/1, Bus Creator/1, Selector9/1  "States_dot_out"
  Actuators Dynamcis/3(Throttle_meas) -> Bus Creator/12  "Throttle"
  Selector9/1 -> Acels actual/1
  Mux1/1 -> Actuators Dynamcis/1(Control_commands)
  Sum1/1 -> Mux1/8
  Sum9/1 -> Mux1/7
  Demux1/6 -> Mux1/6
  Demux1/4 -> Mux1/4
  Demux1/2 -> Mux1/2
  Demux1/1 -> Mux1/1
  Demux1/3 -> Mux1/3
  Demux1/5 -> Mux1/5
  Demux1/7 -> Sum9/1
  Demux1/8 -> Sum1/1
  Model used flag/1 -> Mux5/4
  F16 nlsim nlplant Asymetrical/1 -> Demux/1  "OUTPUTS"
  Mux5/1 -> F16 nlsim nlplant Asymetrical/1  "INPUTS"
  States/1 -> Mux5/1
  Control Comands/1 -> Demux1/1
  Fidelity Flag/1 -> Mux5/3
  Bus Creator/1 -> Leading Edge Flap:Symetric deflection/1(state), Output_bus/1
  Rotation Angles to Direction Cosine Matrix/1 -> Bus Creator/10  "DCM_b"
  Integrate F16 State Derivatives/1 -> Bus Creator/2, Selector/1, Selector2/1, Selector3/1, Selector4/1, Selector5/1  "States_out"
  Actuators Dynamcis/2(Dec_Control_def) -> Mux5/2
  Leading Edge Flap:Symetric deflection/1(delta_lef (deg)) -> Bus Creator1/1, Sum1/2, Sum9/2  "Symetric_LEF_defl"
  Bus Creator1/1 -> Actual control def/1
  Actuators Dynamcis/1(Control Defl Plot) -> Bus Creator1/2  "actual_control_defl"
